simulink library "fuzwiz"  (Simulink 7.4)
settings: Solver=ode45  SolverMode=SingleTasking  StartTime=0.0  StopTime=10.0  RelTol=1e-3
libraries: fuzwiz x2
settings Model: Creator=pascal  LastModifiedBy=rchen

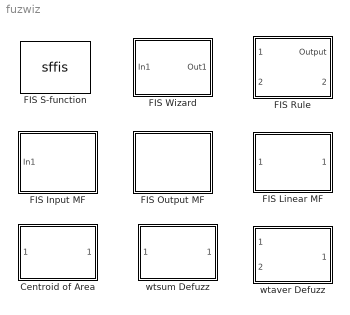
== system fuzwiz ==
  Centroid of Area : Subsystem  mask(COA Defuzzification){range=}
      mask prompts: range "Output Range:"
      mask init:
      | Xdata = linspace(range(1),range(2),101);
      mask Display: disp('COA')
  FIS Input MF : Subsystem  mask(Input MF Eval){fis=, j_in=}
      mask prompts: fis "FIS structure:"; j_in "Input:"
      mask init:
      | fuzwizmask(gcb,fis,j_in)
      mask Display: disp('Input MF')
  FIS Linear MF : Subsystem  mask(Linear Output MF){a=, b=}
      mask prompts: a "Linear Coefficients:"; b "Constant Coefficients:"
      mask Display: disp('Linear MF')
  FIS Output MF : Subsystem  mask(Output MF Eval){fis=, j_out=}
      mask prompts: fis "FIS structure:"; j_out "Output:"
      mask init:
      | fuzwizmask(gcb,fis,j_out)
      mask Display: disp('Output MF')
  FIS Rule : Subsystem  mask(FIS Rule){fis=, j_rule=}
      mask prompts: fis "FIS structure:"; j_rule "Rule:"
      mask init:
      | fuzwizmask(gcb,fis,j_rule)
      mask Display: disp('Rule')
  FIS S-function : S-Function  FunctionName=sffis  Parameters=fis  SFunctionModules=sfsup  EnableBusSupport=off
  FIS Wizard : Subsystem  mask(FIS Wizard){fis=}
      mask prompts: fis "FIS structure:"
      mask init:
      | fuzwizmask(gcb,fis);
      mask Display: disp('FIS')
  wtaver Defuzz : Subsystem
      mask Type: WTAVER Defuzzification
      mask Display: disp('WTAVER')
  wtsum Defuzz : Subsystem
      mask Type: WTSUM Defuzzification
      mask Display: disp('WTSUM')

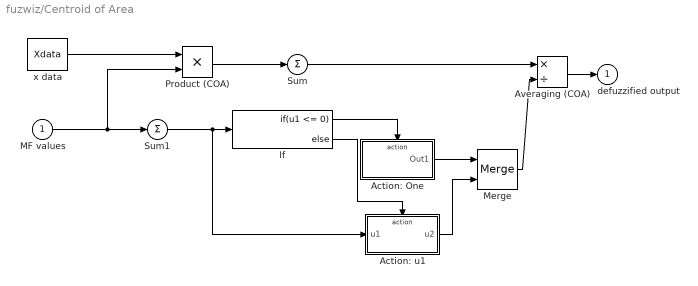
== system fuzwiz/Centroid of Area ==
  MF values : Inport  OutDataType=sfix(16)  OutScaling=2^0
  Action: One : Subsystem  TreatAsAtomicUnit=on
  Action: u1 : Subsystem  TreatAsAtomicUnit=on
  Averaging (COA) : Product  Inputs=*/  OutDataType=sfix(16)  OutScaling=2^0  SaturateOnIntegerOverflow=on  RndMeth=Zero  InputSameDT=on  OutDataTypeStr=Inherit: Same as first input
  If : If  IfExpression=u1 <= 0
  Merge : Merge
  Product (COA) : Product  OutDataType=sfix(16)  OutScaling=2^0  SaturateOnIntegerOverflow=on  RndMeth=Zero  InputSameDT=on  OutDataTypeStr=Inherit: Same as first input
  Sum : Sum  Inputs=+  OutDataType=sfix(16)  OutScaling=2^0  SaturateOnIntegerOverflow=on  InputSameDT=on  OutDataTypeStr=Inherit: Same as first input
  Sum1 : Sum  Inputs=+  OutDataType=sfix(16)  OutScaling=2^0  SaturateOnIntegerOverflow=on  InputSameDT=on  OutDataTypeStr=Inherit: Same as first input
  x data : Constant  Value=Xdata  OutDataType=sfix(16)  OutScaling=2^0
  defuzzified output : Outport  OutDataType=sfix(16)  OutScaling=2^0
  wires:
  Averaging (COA)/1 -> defuzzified output/1
  Sum/1 -> Averaging (COA)/1
  MF values/1 -> Sum1/1, Product (COA)/2
  Product (COA)/1 -> Sum/1
  x data/1 -> Product (COA)/1
  Sum1/1 -> If/1, Action: u1/1(u1)
  If/2 -> Action: u1/Action
  If/1 -> Action: One/Action
  Action: One/1(Out1) -> Merge/1
  Action: u1/1(u2) -> Merge/2
  Merge/1 -> Averaging (COA)/2

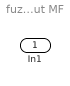
== system fuzwiz/FIS Input MF ==
  In1 : Inport  OutDataType=sfix(16)  OutScaling=2^0

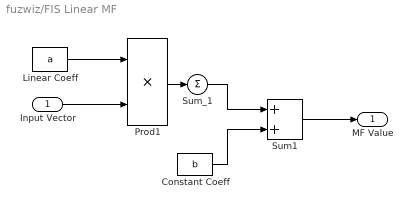
== system fuzwiz/FIS Linear MF ==
  Input Vector : Inport  OutDataType=sfix(16)  OutScaling=2^0
  Constant Coeff : Constant  Value=b  OutDataType=sfix(16)  OutScaling=2^0
  Linear Coeff : Constant  Value=a  OutDataType=sfix(16)  OutScaling=2^0
  Prod1 : Product  OutDataType=sfix(16)  OutScaling=2^0  SaturateOnIntegerOverflow=on  RndMeth=Zero  InputSameDT=on  OutDataTypeStr=Inherit: Same as first input
  Sum1 : Sum  Inputs=2  OutDataType=sfix(16)  OutScaling=2^0  SaturateOnIntegerOverflow=on  InputSameDT=on  OutDataTypeStr=Inherit: Same as first input
  Sum_1 : Sum  Inputs=1  OutDataType=sfix(16)  OutScaling=2^0  SaturateOnIntegerOverflow=on  InputSameDT=on  OutDataTypeStr=Inherit: Same as first input
  MF Value : Outport  OutDataType=sfix(16)  OutScaling=2^0
  wires:
  Linear Coeff/1 -> Prod1/1
  Prod1/1 -> Sum_1/1
  Sum_1/1 -> Sum1/1
  Constant Coeff/1 -> Sum1/2
  Input Vector/1 -> Prod1/2
  Sum1/1 -> MF Value/1

== system fuzwiz/FIS Output MF ==

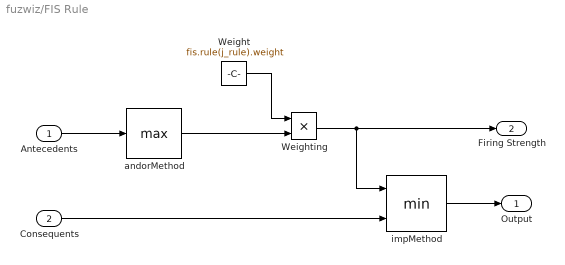
== system fuzwiz/FIS Rule ==
  Antecedents : Inport  OutDataType=sfix(16)  OutScaling=2^0
  Consequents : Inport  Port=2  OutDataType=sfix(16)  OutScaling=2^0
  Weight : Constant  Value=fis.rule(j_rule).weight  OutDataType=sfix(16)  OutScaling=2^0
  Weighting : Product  OutDataType=sfix(16)  OutScaling=2^0  SaturateOnIntegerOverflow=on  RndMeth=Zero  InputSameDT=on  OutDataTypeStr=Inherit: Same as first input
  andorMethod : MinMax  Function=max  OutDataType=sfix(16)  OutScaling=2^0  SaturateOnIntegerOverflow=on  InputSameDT=on
  impMethod : MinMax  Inputs=2  OutDataType=sfix(16)  OutScaling=2^0  SaturateOnIntegerOverflow=on  InputSameDT=on
  Output : Outport  OutDataType=sfix(16)  OutScaling=2^0
  Firing Strength : Outport  Port=2  OutDataType=sfix(16)  OutScaling=2^0
  wires:
  Antecedents/1 -> andorMethod/1
  andorMethod/1 -> Weighting/2
  Weight/1 -> Weighting/1
  Consequents/1 -> impMethod/2
  Weighting/1 -> impMethod/1, Firing Strength/1
  impMethod/1 -> Output/1

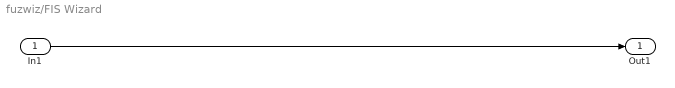
== system fuzwiz/FIS Wizard ==
  In1 : Inport  OutDataType=sfix(16)  OutScaling=2^0
  Out1 : Outport  OutDataType=sfix(16)  OutScaling=2^0
  wires:
  In1/1 -> Out1/1

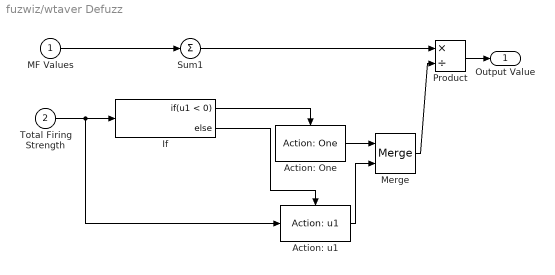
== system fuzwiz/wtaver Defuzz ==
  MF Values : Inport  OutDataType=sfix(16)  OutScaling=2^0
  Total Firing Strength : Inport  Port=2  OutDataType=sfix(16)  OutScaling=2^0
  Action: One : fuzwiz/Centroid of Area/Action: One  SystemSampleTime=-1
  Action: u1 : fuzwiz/Centroid of Area/Action: u1  SystemSampleTime=-1
  If : If  IfExpression=u1 < 0
  Merge : Merge
  Product : Product  Inputs=*/  OutDataType=sfix(16)  OutScaling=2^0  SaturateOnIntegerOverflow=on  RndMeth=Zero  InputSameDT=on  OutDataTypeStr=Inherit: Same as first input
  Sum1 : Sum  Inputs=1  OutDataType=sfix(16)  OutScaling=2^0  SaturateOnIntegerOverflow=on  InputSameDT=on  OutDataTypeStr=Inherit: Same as first input
  Output Value : Outport  OutDataType=sfix(16)  OutScaling=2^0
  wires:
  MF Values/1 -> Sum1/1
  Sum1/1 -> Product/1
  Product/1 -> Output Value/1
  Total Firing Strength/1 -> If/1, Action: u1/1
  If/1 -> Action: One/Action
  If/2 -> Action: u1/Action
  Action: One/1 -> Merge/1
  Action: u1/1 -> Merge/2
  Merge/1 -> Product/2

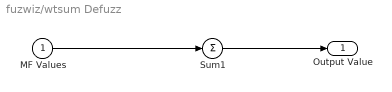
== system fuzwiz/wtsum Defuzz ==
  MF Values : Inport  OutDataType=sfix(16)  OutScaling=2^0
  Sum1 : Sum  Inputs=1  OutDataType=sfix(16)  OutScaling=2^0  SaturateOnIntegerOverflow=on  InputSameDT=on  OutDataTypeStr=Inherit: Same as first input
  Output Value : Outport  OutDataType=sfix(16)  OutScaling=2^0
  wires:
  MF Values/1 -> Sum1/1
  Sum1/1 -> Output Value/1

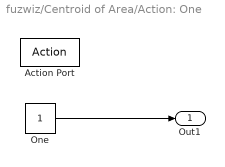
== system fuzwiz/Centroid of Area/Action: One ==
  Action Port : ActionPort  ActionType=then
  One : Constant  OutDataType=sfix(16)  OutScaling=2^0
  Out1 : Outport  OutDataType=sfix(16)  OutScaling=2^0  InitialOutput=0
  wires:
  One/1 -> Out1/1

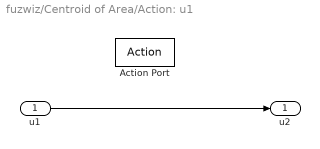
== system fuzwiz/Centroid of Area/Action: u1 ==
  u1 : Inport  OutDataType=sfix(16)  OutScaling=2^0
  Action Port : ActionPort  ActionType=else
  u2 : Outport  OutDataType=sfix(16)  OutScaling=2^0
  wires:
  u1/1 -> u2/1
